simulink model "RoboSoccerSim"  (R2022b)
settings: Solver=ode4  StartTime=0.0  StopTime=inf  FixedStep=0.01  RelTol=1e-3
libraries: dspindex x20
(part 2 of 2)

== stateflow chart RoboSoccerSim/Robot Team Clients 2 (Away)/Subsystem/Away Player Strategy 3 ==
  state InitialState
    en,du:
    if gameSituation.kickConfirmation == true
    robotCommand.kick = false;
    end
    id = 3; % Team1(Home) Robot 1
    shootDistThres = 2500;
    kickableAreaRadius = 20;
    homeGoalPose = [5000, 0];
    awayGoalPose = [-5000, 0];
    homeAttackPositions = [[-2500, 0, 180]; [-1500, 2000, 180]; [-1500, -2000, 180]; [2000, 0, 180]];
    homeDefendPositions = [[1000, 0, 180]; [3000, 2000, 180]; [3000, -2000, 180]; [3500, 0, 180]];
  state ROBOT 1 [group]
    (Strategy for robot 1~3)
  state Attack
    en,du:
    %%calculate the distance to the goal
    teamDistToGoal = [0 0 0 0];
    for idx=1:1:4
    teamDistToGoal(idx) = distTo(gameSituation.robotCurrentPose(idx,1:2), awayGoalPose);
    end
    distToGoal1 = distTo(gameSituation.robotCurrentPose(id,1:2), awayGoalPose);
    %calculate the distance to the ball
    teamDistToBall = [0 0 0 0];
    for idx=1:1:4
    teamDistToBall(idx) = distTo(gameSituation.robotCurrentPose(idx,1:2), ...
    gameSituation.ballCurrentPose(1:2));
    end
    distToBall = distTo(gameSituation.robotCurrentPose(id,1:2), ...
    gameSituation.ballCurrentPose(1:2));
  state Defend
    en,du:
    %%calculate the distance to the home goal
    teamDistToOwnGoal = [0 0 0 0];
    for idx=1:1:4
    teamDistToOwnGoal(idx) = distTo(gameSituation.robotCurrentPose(idx,1:2), homeGoalPose);
    end
    distToOwnGoal = distTo(gameSituation.robotCurrentPose(id,1:2), homeGoalPose);
    for idx=1:1:4
    teamDistToBall(idx) = distTo(gameSituation.robotCurrentPose(idx,1:2), ...
    gameSituation.ballCurrentPose(1:2));
    end
    distToBall = distTo(gameSituation.robotCurrentPose(id,1:2), ...
    gameSituation.ballCurrentPose(1:2));
  state Position
    en,du:
    playerAttackPosition = homeAttackPositions(id, :);
    kickPower = 1;
    kickState = false;
    desiredPosition = playerAttackPosition;
    isdone = true;
  state Shoot
    en,du:
    angleBallGoal = atan2d(awayGoalPose(2) - gameSituation.ballCurrentPose(2), ...
    awayGoalPose(1) - gameSituation.ballCurrentPose(1));
    kickPower = 100;
    kickState = true;
    kickDirection = angleBallGoal;
    xPosition= gameSituation.ballCurrentPose(1) + cosd(180 - angleBallGoal) * kickableAreaRadius;
    yPosition = gameSituation.ballCurrentPose(2) + sind(180 - angleBallGoal) * kickableAreaRadius;
    desiredPosition = [xPosition, yPosition, kickDirection];
    isdone = true;
  state Pass
    en,du:
    [minval,minidx] = min(teamDistToGoal)
    angleBallPlayer = atan2d(gameSituation.robotCurrentPose(minidx, 2) - gameSituation.ballCurrentPose(2), ...
    gameSituation.robotCurrentPose(minidx, 1) - gameSituation.ballCurrentPose(1));
    kickPower = 66;
    kickState = true;
    kickDirection = angleBallPlayer;
    xPosition= gameSituation.ballCurrentPose(1) + cosd(180 - angleBallGoal) * kickableAreaRadius;
    yPosition = gameSituation.ballCurrentPose(2) + sind(180 - angleBallGoal) * kickableAreaRadius;
    desiredPosition = [xPosition, yPosition, kickDirection];
    isdone = true;
  state Dribble
    en,du:
    angleBallGoal = atan2d(awayGoalPose(2) - gameSituation.ballCurrentPose(2), ...
    awayGoalPose(1) - gameSituation.ballCurrentPose(1));
    kickPower = 10;
    %%should be designed as the kickPower = kickPowerCofficent * 100
    %%kickPowerCofficieant should also be calculated by distance
    kickState = true;
    kickDirection = angleBallGoal;
    xPosition= gameSituation.ballCurrentPose(1) + cosd(180 - angleBallGoal) * kickableAreaRadius;
    yPosition = gameSituation.ballCurrentPose(2) + sind(180 - angleBallGoal) * kickableAreaRadius;
    desiredPosition = [xPosition, yPosition, kickDirection];
    isdone = true;
  state Intercept
    en,du:
    angleBallGoal = atan2d(awayGoalPose(2) - gameSituation.ballCurrentPose(2), ...
    awayGoalPose(1) - gameSituation.ballCurrentPose(1));
    kickPower = 50;
    kickState = true;
    kickDirection = angleBallGoal;
    xPosition= gameSituation.ballCurrentPose(1) + cosd(180 - angleBallGoal) * kickableAreaRadius;
    yPosition = gameSituation.ballCurrentPose(2) + sind(180 - angleBallGoal) * kickableAreaRadius;
    desiredPosition = [xPosition, yPosition, kickDirection];
    isdone = true;
  state Formation
    en,du:
    playerDefendPosition = homeDefendPositions(id, :);
    kickPower = 1;
    kickState = false;
    desiredPosition = playerDefendPosition;
    isdone = true;
  state Kick
    state MoveTo1
      en,du:
      isdone = false;
      robotCommand.robotDestinationPose = desiredPosition;
      distToBall = distTo(gameSituation.robotCurrentPose(id,1:2), ...
      gameSituation.ballCurrentPose(1:2));
    state KickTo
      en,du:
      robotCommand.kick = kickState;
      robotCommand.kickProperty = kickPower;
      isdone = true;
    MoveTo1 -> KickTo [order 1] : [distToBall <= kickableAreaRadius+5]
  MoveTo1 -> InitialState [order 2] : [after(2,sec)]
  KickTo -> InitialState : [after(5,sec)]
  (default) -> InitialState
  InitialState -> Attack [order 2] : [gameSituation.ballLastCommandBy(1) == 2]
  InitialState -> Defend [order 1] : [gameSituation.ballLastCommandBy(1) == 1]
  Attack -> Position [order 1] : [distToBall ~= min(teamDistToBall)]
  Defend -> Intercept [order 1] : [distToBall ~= max(teamDistToBall)]
  Defend -> Formation [order 2] : [distToBall == max(teamDistToBall)]
  Attack -> Pass [order 3] : [distToGoal1 ~= min(teamDistToGoal)&& distToBall == min(teamDistToBall)]
  Attack -> Dribble [order 4] : [distToBall == min(teamDistToBall) && distToGoal1 == min(teamDistToGoal) && distToGoal1 > shootDistThres]
  Attack -> Shoot [order 2] : [distToBall == min(teamDistToBall) && distToGoal1 == min(teamDistToGoal) && distToGoal1 < shootDistThres]
  Intercept -> MoveTo1 : [isdone]
  Formation -> MoveTo1 : [isdone]
  Pass -> MoveTo1 : [isdone]
  Dribble -> MoveTo1 : [isdone]
  Shoot -> MoveTo1 : [isdone]
  Position -> MoveTo1 : [isdone]
  data: robotPosition function_input; goalPosition function_input; dist function_output; awayGoalPose local =[0 0]; homeGoalPose local =[0 0]; id local =1; idx local; angleBallGoal local =0; desiredPosition local =[0 0 0]; distToOwnGoal local =0; kickDirection local =0; kickPower local =0; kickState local =false; minidx local; playerDefendPosition local =[0 0 0]; teamDistToGoal local =[0 0 0 0]; teamDistToOwnGoal local =[0 0 0 0]; minval local; isdone local boolean =false; playerAttackPosition local =[0 0 0]; shootDistThres local =0; gameSituation input Bus: gameSituation; kickableAreaRadius local =0; distToGoal1 local =0; angleBallPlayer local =0; robotCommand output Bus: robotCommand; distToBall local =0; teamDistToBall local =[0 0 0 0]; homeAttackPositions local =[0 0 0;0 0 0;0 0 0;0 0 0]; homeDefendPositions local =[0 0 0;0 0 0;0 0 0;0 0 0]; xPosition local; yPosition local
  function dist = distTo(robotPosition,goalPosition):
    | function dist = distTo(robotPosition,goalPosition)
    |     dist = norm(robotPosition - goalPosition);
    | end

== stateflow chart RoboSoccerSim/Robot Team Clients 1 (Home)/Subsystem/Home Player Strategy 1 ==
  state InitialState
    en,du:
    if gameSituation.kickConfirmation == true
    robotCommand.kick = false;
    end
    id = 1; % Team1(Home) Robot 1
    shootDistThres = 2500;
    kickableAreaRadius = 20;
    homeGoalPose = [-5000, 0];
    awayGoalPose = [5000, 0];
    homeAttackPositions = [[2500, 0, 0]; [1500, 2000, 0]; [1500, -2000, 0]; [-2000, 0, 0]];
    homeDefendPositions = [[-1000, 0, 0]; [-3000, 2000, 0]; [-3000, -2000, 0]; [-3500, 0, 0]];
  state ROBOT 1 [group]
    (Strategy for robot 1~3)
  state Attack
    en,du:
    %%calculate the distance to the goal
    teamDistToGoal = [0 0 0 0];
    for idx=1:1:4
    teamDistToGoal(idx) = distTo(gameSituation.robotCurrentPose(idx,1:2), awayGoalPose);
    end
    distToGoal1 = distTo(gameSituation.robotCurrentPose(id,1:2), awayGoalPose);
    %calculate the distance to the ball
    teamDistToBall = [0 0 0 0];
    for idx=1:1:4
    teamDistToBall(idx) = distTo(gameSituation.robotCurrentPose(idx,1:2), ...
    gameSituation.ballCurrentPose(1:2));
    end
    distToBall = distTo(gameSituation.robotCurrentPose(id,1:2), ...
    gameSituation.ballCurrentPose(1:2));
  state Defend
    en,du:
    %%calculate the distance to the home goal
    teamDistToOwnGoal = [0 0 0 0];
    for idx=1:1:4
    teamDistToOwnGoal(idx) = distTo(gameSituation.robotCurrentPose(idx,1:2), homeGoalPose);
    end
    distToOwnGoal = distTo(gameSituation.robotCurrentPose(id,1:2), homeGoalPose);
    for idx=1:1:4
    teamDistToBall(idx) = distTo(gameSituation.robotCurrentPose(idx,1:2), ...
    gameSituation.ballCurrentPose(1:2));
    end
    distToBall = distTo(gameSituation.robotCurrentPose(id,1:2), ...
    gameSituation.ballCurrentPose(1:2));
  state Position
    en,du:
    playerAttackPosition = homeAttackPositions(id, :);
    kickPower = 1;
    kickState = false;
    desiredPosition = playerAttackPosition;
    isdone = true;
  state Shoot
    en,du:
    angleBallGoal = atan2d(awayGoalPose(2) - gameSituation.ballCurrentPose(2), ...
    awayGoalPose(1) - gameSituation.ballCurrentPose(1));
    kickPower = 100;
    kickState = true;
    kickDirection = angleBallGoal;
    xPosition= gameSituation.ballCurrentPose(1) + cosd(180 - angleBallGoal) * kickableAreaRadius;
    yPosition = gameSituation.ballCurrentPose(2) + sind(180 - angleBallGoal) * kickableAreaRadius;
    desiredPosition = [xPosition, yPosition, kickDirection];
    isdone = true;
  state Pass
    en,du:
    [minval,minidx] = min(teamDistToGoal)
    angleBallPlayer = atan2d(gameSituation.robotCurrentPose(minidx, 2) - gameSituation.ballCurrentPose(2), ...
    gameSituation.robotCurrentPose(minidx, 1) - gameSituation.ballCurrentPose(1));
    kickPower = 66;
    kickState = true;
    kickDirection = angleBallPlayer;
    xPosition= gameSituation.ballCurrentPose(1) + cosd(180 - angleBallGoal) * kickableAreaRadius;
    yPosition = gameSituation.ballCurrentPose(2) + sind(180 - angleBallGoal) * kickableAreaRadius;
    desiredPosition = [xPosition, yPosition, kickDirection];
    isdone = true;
  state Dribble
    en,du:
    angleBallGoal = atan2d(awayGoalPose(2) - gameSituation.ballCurrentPose(2), ...
    awayGoalPose(1) - gameSituation.ballCurrentPose(1));
    kickPower = 20;
    %%should be designed as the kickPower = kickPowerCofficent * 100
    %%kickPowerCofficieant should also be calculated by distance
    kickState = true;
    kickDirection = angleBallGoal;
    xPosition= gameSituation.ballCurrentPose(1) + cosd(180 - angleBallGoal) * kickableAreaRadius;
    yPosition = gameSituation.ballCurrentPose(2) + sind(180 - angleBallGoal) * kickableAreaRadius;
    desiredPosition = [xPosition, yPosition, kickDirection];
    isdone = true;
  state Intercept
    en,du:
    angleBallGoal = atan2d(awayGoalPose(2) - gameSituation.ballCurrentPose(2), ...
    awayGoalPose(1) - gameSituation.ballCurrentPose(1));
    kickPower = 50;
    kickState = true;
    kickDirection = angleBallGoal;
    xPosition= gameSituation.ballCurrentPose(1) + cosd(180 - angleBallGoal) * kickableAreaRadius;
    yPosition = gameSituation.ballCurrentPose(2) + sind(180 - angleBallGoal) * kickableAreaRadius;
    desiredPosition = [xPosition, yPosition, kickDirection];
    isdone = true;
  state Formation
    en,du:
    playerDefendPosition = homeDefendPositions(id, :);
    kickPower = 1;
    kickState = false;
    desiredPosition = playerDefendPosition;
    isdone = true;
  state Kick
    state MoveTo1
      en,du:
      isdone = false;
      robotCommand.robotDestinationPose = desiredPosition;
      distToBall = distTo(gameSituation.robotCurrentPose(id,1:2), ...
      gameSituation.ballCurrentPose(1:2));
    state KickTo
      en,du:
      robotCommand.kick = kickState;
      robotCommand.kickProperty = kickPower;
      isdone = true;
    MoveTo1 -> KickTo [order 1] : [distToBall <= kickableAreaRadius+5]
  MoveTo1 -> InitialState [order 2] : [after(2,sec)]
  KickTo -> InitialState : [after(5,sec)]
  (default) -> InitialState
  InitialState -> Attack [order 2] : [gameSituation.ballLastCommandBy(1) == 1]
  InitialState -> Defend [order 1] : [gameSituation.ballLastCommandBy(1) == 2]
  Attack -> Position [order 1] : [distToBall ~= min(teamDistToBall)]
  Defend -> Intercept [order 1] : [distToBall ~= max(teamDistToBall)]
  Defend -> Formation [order 2] : [distToBall == max(teamDistToBall)]
  Attack -> Pass [order 3] : [distToGoal1 ~= min(teamDistToGoal)&& distToBall == min(teamDistToBall)]
  Attack -> Dribble [order 4] : [distToBall == min(teamDistToBall) && distToGoal1 == min(teamDistToGoal) && distToGoal1 > shootDistThres]
  Attack -> Shoot [order 2] : [distToBall == min(teamDistToBall) && distToGoal1 == min(teamDistToGoal) && distToGoal1 < shootDistThres]
  Intercept -> MoveTo1 : [isdone]
  Formation -> MoveTo1 : [isdone]
  Pass -> MoveTo1 : [isdone]
  Dribble -> MoveTo1 : [isdone]
  Shoot -> MoveTo1 : [isdone]
  Position -> MoveTo1 : [isdone]
  data: robotPosition function_input; goalPosition function_input; dist function_output; awayGoalPose local =[0 0]; homeGoalPose local =[0 0]; id local =1; idx local; angleBallGoal local =0; desiredPosition local =[0 0 0]; distToOwnGoal local =0; kickDirection local =0; kickPower local =0; kickState local =false; minidx local; playerDefendPosition local =[0 0 0]; teamDistToGoal local =[0 0 0 0]; teamDistToOwnGoal local =[0 0 0 0]; minval local; isdone local boolean =false; playerAttackPosition local =[0 0 0]; shootDistThres local =0; gameSituation input Bus: gameSituation; kickableAreaRadius local =0; distToGoal1 local =0; angleBallPlayer local =0; robotCommand output Bus: robotCommand; distToBall local =0; teamDistToBall local =[0 0 0 0]; homeAttackPositions local =[0 0 0;0 0 0;0 0 0;0 0 0]; homeDefendPositions local =[0 0 0;0 0 0;0 0 0;0 0 0]; xPosition local; yPosition local
  function dist = distTo(robotPosition,goalPosition):
    | function dist = distTo(robotPosition,goalPosition)
    |     dist = norm(robotPosition - goalPosition);
    | end

== stateflow chart RoboSoccerSim/Robot Team Clients 1 (Home)/Subsystem/Home Player Strategy 2 ==
  state InitialState
    en,du:
    if gameSituation.kickConfirmation == true
    robotCommand.kick = false;
    end
    id = 2; % Team1(Home) Robot 1
    shootDistThres = 2500;
    kickableAreaRadius = 20;
    homeGoalPose = [-5000, 0];
    awayGoalPose = [5000, 0];
    homeAttackPositions = [[2500, 0, 0]; [1500, 2000, 0]; [1500, -2000, 0]; [-2000, 0, 0]];
    homeDefendPositions = [[-1000, 0, 0]; [-3000, 2000, 0]; [-3000, -2000, 0]; [-3500, 0, 0]];
  state ROBOT 1 [group]
    (Strategy for robot 1~3)
  state Attack
    en,du:
    %%calculate the distance to the goal
    teamDistToGoal = [0 0 0 0];
    for idx=1:1:4
    teamDistToGoal(idx) = distTo(gameSituation.robotCurrentPose(idx,1:2), awayGoalPose);
    end
    distToGoal1 = distTo(gameSituation.robotCurrentPose(id,1:2), awayGoalPose);
    %calculate the distance to the ball
    teamDistToBall = [0 0 0 0];
    for idx=1:1:4
    teamDistToBall(idx) = distTo(gameSituation.robotCurrentPose(idx,1:2), ...
    gameSituation.ballCurrentPose(1:2));
    end
    distToBall = distTo(gameSituation.robotCurrentPose(id,1:2), ...
    gameSituation.ballCurrentPose(1:2));
  state Defend
    en,du:
    %%calculate the distance to the home goal
    teamDistToOwnGoal = [0 0 0 0];
    for idx=1:1:4
    teamDistToOwnGoal(idx) = distTo(gameSituation.robotCurrentPose(idx,1:2), homeGoalPose);
    end
    distToOwnGoal = distTo(gameSituation.robotCurrentPose(id,1:2), homeGoalPose);
    for idx=1:1:4
    teamDistToBall(idx) = distTo(gameSituation.robotCurrentPose(idx,1:2), ...
    gameSituation.ballCurrentPose(1:2));
    end
    distToBall = distTo(gameSituation.robotCurrentPose(id,1:2), ...
    gameSituation.ballCurrentPose(1:2));
  state Position
    en,du:
    playerAttackPosition = homeAttackPositions(id, :);
    kickPower = 1;
    kickState = false;
    desiredPosition = playerAttackPosition;
    isdone = true;
  state Shoot
    en,du:
    angleBallGoal = atan2d(awayGoalPose(2) - gameSituation.ballCurrentPose(2), ...
    awayGoalPose(1) - gameSituation.ballCurrentPose(1));
    kickPower = 100;
    kickState = true;
    kickDirection = angleBallGoal;
    xPosition= gameSituation.ballCurrentPose(1) + cosd(180 - angleBallGoal) * kickableAreaRadius;
    yPosition = gameSituation.ballCurrentPose(2) + sind(180 - angleBallGoal) * kickableAreaRadius;
    desiredPosition = [xPosition, yPosition, kickDirection];
    isdone = true;
  state Pass
    en,du:
    [minval,minidx] = min(teamDistToGoal)
    angleBallPlayer = atan2d(gameSituation.robotCurrentPose(minidx, 2) - gameSituation.ballCurrentPose(2), ...
    gameSituation.robotCurrentPose(minidx, 1) - gameSituation.ballCurrentPose(1));
    kickPower = 66;
    kickState = true;
    kickDirection = angleBallPlayer;
    xPosition= gameSituation.ballCurrentPose(1) + cosd(180 - angleBallGoal) * kickableAreaRadius;
    yPosition = gameSituation.ballCurrentPose(2) + sind(180 - angleBallGoal) * kickableAreaRadius;
    desiredPosition = [xPosition, yPosition, kickDirection];
    isdone = true;
  state Dribble
    en,du:
    angleBallGoal = atan2d(awayGoalPose(2) - gameSituation.ballCurrentPose(2), ...
    awayGoalPose(1) - gameSituation.ballCurrentPose(1));
    kickPower = 20;
    %%should be designed as the kickPower = kickPowerCofficent * 100
    %%kickPowerCofficieant should also be calculated by distance
    kickState = true;
    kickDirection = angleBallGoal;
    xPosition= gameSituation.ballCurrentPose(1) + cosd(180 - angleBallGoal) * kickableAreaRadius;
    yPosition = gameSituation.ballCurrentPose(2) + sind(180 - angleBallGoal) * kickableAreaRadius;
    desiredPosition = [xPosition, yPosition, kickDirection];
    isdone = true;
  state Intercept
    en,du:
    angleBallGoal = atan2d(awayGoalPose(2) - gameSituation.ballCurrentPose(2), ...
    awayGoalPose(1) - gameSituation.ballCurrentPose(1));
    kickPower = 50;
    kickState = true;
    kickDirection = angleBallGoal;
    xPosition= gameSituation.ballCurrentPose(1) + cosd(180 - angleBallGoal) * kickableAreaRadius;
    yPosition = gameSituation.ballCurrentPose(2) + sind(180 - angleBallGoal) * kickableAreaRadius;
    desiredPosition = [xPosition, yPosition, kickDirection];
    isdone = true;
  state Formation
    en,du:
    playerDefendPosition = homeDefendPositions(id, :);
    kickPower = 1;
    kickState = false;
    desiredPosition = playerDefendPosition;
    isdone = true;
  state Kick
    state MoveTo1
      en,du:
      isdone = false;
      robotCommand.robotDestinationPose = desiredPosition;
      distToBall = distTo(gameSituation.robotCurrentPose(id,1:2), ...
      gameSituation.ballCurrentPose(1:2));
    state KickTo
      en,du:
      robotCommand.kick = kickState;
      robotCommand.kickProperty = kickPower;
      isdone = true;
    MoveTo1 -> KickTo [order 1] : [distToBall <= kickableAreaRadius+5]
  MoveTo1 -> InitialState [order 2] : [after(2,sec)]
  KickTo -> InitialState : [after(5,sec)]
  (default) -> InitialState
  InitialState -> Attack [order 2] : [gameSituation.ballLastCommandBy(1) == 1]
  InitialState -> Defend [order 1] : [gameSituation.ballLastCommandBy(1) == 2]
  Attack -> Position [order 1] : [distToBall ~= min(teamDistToBall)]
  Defend -> Intercept [order 1] : [distToBall ~= max(teamDistToBall)]
  Defend -> Formation [order 2] : [distToBall == max(teamDistToBall)]
  Attack -> Pass [order 3] : [distToGoal1 ~= min(teamDistToGoal)&& distToBall == min(teamDistToBall)]
  Attack -> Dribble [order 4] : [distToBall == min(teamDistToBall) && distToGoal1 == min(teamDistToGoal) && distToGoal1 > shootDistThres]
  Attack -> Shoot [order 2] : [distToBall == min(teamDistToBall) && distToGoal1 == min(teamDistToGoal) && distToGoal1 < shootDistThres]
  Intercept -> MoveTo1 : [isdone]
  Formation -> MoveTo1 : [isdone]
  Pass -> MoveTo1 : [isdone]
  Dribble -> MoveTo1 : [isdone]
  Shoot -> MoveTo1 : [isdone]
  Position -> MoveTo1 : [isdone]
  data: robotPosition function_input; goalPosition function_input; dist function_output; awayGoalPose local =[0 0]; homeGoalPose local =[0 0]; id local =1; idx local; angleBallGoal local =0; desiredPosition local =[0 0 0]; distToOwnGoal local =0; kickDirection local =0; kickPower local =0; kickState local =false; minidx local; playerDefendPosition local =[0 0 0]; teamDistToGoal local =[0 0 0 0]; teamDistToOwnGoal local =[0 0 0 0]; minval local; isdone local boolean =false; playerAttackPosition local =[0 0 0]; shootDistThres local =0; gameSituation input Bus: gameSituation; kickableAreaRadius local =0; distToGoal1 local =0; angleBallPlayer local =0; robotCommand output Bus: robotCommand; distToBall local =0; teamDistToBall local =[0 0 0 0]; homeAttackPositions local =[0 0 0;0 0 0;0 0 0;0 0 0]; homeDefendPositions local =[0 0 0;0 0 0;0 0 0;0 0 0]; xPosition local; yPosition local
  function dist = distTo(robotPosition,goalPosition):
    | function dist = distTo(robotPosition,goalPosition)
    |     dist = norm(robotPosition - goalPosition);
    | end

== stateflow chart RoboSoccerSim/Robot Team Clients 1 (Home)/Subsystem/Home Player Strategy 3 ==
  state InitialState
    en,du:
    if gameSituation.kickConfirmation == true
    robotCommand.kick = false;
    end
    id = 3; % Team1(Home) Robot 1
    shootDistThres = 2500;
    kickableAreaRadius = 20;
    homeGoalPose = [-5000, 0];
    awayGoalPose = [5000, 0];
    homeAttackPositions = [[2500, 0, 0]; [1500, 2000, 0]; [1500, -2000, 0]; [-2000, 0, 0]];
    homeDefendPositions = [[-1000, 0, 0]; [-3000, 2000, 0]; [-3000, -2000, 0]; [-3500, 0, 0]];
  state ROBOT 1 [group]
    (Strategy for robot 1~3)
  state Attack
    en,du:
    %%calculate the distance to the goal
    teamDistToGoal = [0 0 0 0];
    for idx=1:1:4
    teamDistToGoal(idx) = distTo(gameSituation.robotCurrentPose(idx,1:2), awayGoalPose);
    end
    distToGoal1 = distTo(gameSituation.robotCurrentPose(id,1:2), awayGoalPose);
    %calculate the distance to the ball
    teamDistToBall = [0 0 0 0];
    for idx=1:1:4
    teamDistToBall(idx) = distTo(gameSituation.robotCurrentPose(idx,1:2), ...
    gameSituation.ballCurrentPose(1:2));
    end
    distToBall = distTo(gameSituation.robotCurrentPose(id,1:2), ...
    gameSituation.ballCurrentPose(1:2));
  state Defend
    en,du:
    %%calculate the distance to the home goal
    teamDistToOwnGoal = [0 0 0 0];
    for idx=1:1:4
    teamDistToOwnGoal(idx) = distTo(gameSituation.robotCurrentPose(idx,1:2), homeGoalPose);
    end
    distToOwnGoal = distTo(gameSituation.robotCurrentPose(id,1:2), homeGoalPose);
    for idx=1:1:4
    teamDistToBall(idx) = distTo(gameSituation.robotCurrentPose(idx,1:2), ...
    gameSituation.ballCurrentPose(1:2));
    end
    distToBall = distTo(gameSituation.robotCurrentPose(id,1:2), ...
    gameSituation.ballCurrentPose(1:2));
  state Position
    en,du:
    playerAttackPosition = homeAttackPositions(id, :);
    kickPower = 1;
    kickState = false;
    desiredPosition = playerAttackPosition;
    isdone = true;
  state Shoot
    en,du:
    angleBallGoal = atan2d(awayGoalPose(2) - gameSituation.ballCurrentPose(2), ...
    awayGoalPose(1) - gameSituation.ballCurrentPose(1));
    kickPower = 100;
    kickState = true;
    kickDirection = angleBallGoal;
    xPosition= gameSituation.ballCurrentPose(1) + cosd(180 - angleBallGoal) * kickableAreaRadius;
    yPosition = gameSituation.ballCurrentPose(2) + sind(180 - angleBallGoal) * kickableAreaRadius;
    desiredPosition = [xPosition, yPosition, kickDirection];
    isdone = true;
  state Pass
    en,du:
    [minval,minidx] = min(teamDistToGoal)
    angleBallPlayer = atan2d(gameSituation.robotCurrentPose(minidx, 2) - gameSituation.ballCurrentPose(2), ...
    gameSituation.robotCurrentPose(minidx, 1) - gameSituation.ballCurrentPose(1));
    kickPower = 66;
    kickState = true;
    kickDirection = angleBallPlayer;
    xPosition= gameSituation.ballCurrentPose(1) + cosd(180 - angleBallGoal) * kickableAreaRadius;
    yPosition = gameSituation.ballCurrentPose(2) + sind(180 - angleBallGoal) * kickableAreaRadius;
    desiredPosition = [xPosition, yPosition, kickDirection];
    isdone = true;
  state Dribble
    en,du:
    angleBallGoal = atan2d(awayGoalPose(2) - gameSituation.ballCurrentPose(2), ...
    awayGoalPose(1) - gameSituation.ballCurrentPose(1));
    kickPower = 20;
    %%should be designed as the kickPower = kickPowerCofficent * 100
    %%kickPowerCofficieant should also be calculated by distance
    kickState = true;
    kickDirection = angleBallGoal;
    xPosition= gameSituation.ballCurrentPose(1) + cosd(180 - angleBallGoal) * kickableAreaRadius;
    yPosition = gameSituation.ballCurrentPose(2) + sind(180 - angleBallGoal) * kickableAreaRadius;
    desiredPosition = [xPosition, yPosition, kickDirection];
    isdone = true;
  state Intercept
    en,du:
    angleBallGoal = atan2d(awayGoalPose(2) - gameSituation.ballCurrentPose(2), ...
    awayGoalPose(1) - gameSituation.ballCurrentPose(1));
    kickPower = 50;
    kickState = true;
    kickDirection = angleBallGoal;
    xPosition= gameSituation.ballCurrentPose(1) + cosd(180 - angleBallGoal) * kickableAreaRadius;
    yPosition = gameSituation.ballCurrentPose(2) + sind(180 - angleBallGoal) * kickableAreaRadius;
    desiredPosition = [xPosition, yPosition, kickDirection];
    isdone = true;
  state Formation
    en,du:
    playerDefendPosition = homeDefendPositions(id, :);
    kickPower = 1;
    kickState = false;
    desiredPosition = playerDefendPosition;
    isdone = true;
  state Kick
    state MoveTo1
      en,du:
      isdone = false;
      robotCommand.robotDestinationPose = desiredPosition;
      distToBall = distTo(gameSituation.robotCurrentPose(id,1:2), ...
      gameSituation.ballCurrentPose(1:2));
    state KickTo
      en,du:
      robotCommand.kick = kickState;
      robotCommand.kickProperty = kickPower;
      isdone = true;
    MoveTo1 -> KickTo [order 1] : [distToBall <= kickableAreaRadius+5]
  MoveTo1 -> InitialState [order 2] : [after(2,sec)]
  KickTo -> InitialState : [after(5,sec)]
  (default) -> InitialState
  InitialState -> Attack [order 2] : [gameSituation.ballLastCommandBy(1) == 1]
  InitialState -> Defend [order 1] : [gameSituation.ballLastCommandBy(1) == 2]
  Attack -> Position [order 1] : [distToBall ~= min(teamDistToBall)]
  Defend -> Intercept [order 1] : [distToBall ~= max(teamDistToBall)]
  Defend -> Formation [order 2] : [distToBall == max(teamDistToBall)]
  Attack -> Pass [order 3] : [distToGoal1 ~= min(teamDistToGoal)&& distToBall == min(teamDistToBall)]
  Attack -> Dribble [order 4] : [distToBall == min(teamDistToBall) && distToGoal1 == min(teamDistToGoal) && distToGoal1 > shootDistThres]
  Attack -> Shoot [order 2] : [distToBall == min(teamDistToBall) && distToGoal1 == min(teamDistToGoal) && distToGoal1 < shootDistThres]
  Intercept -> MoveTo1 : [isdone]
  Formation -> MoveTo1 : [isdone]
  Pass -> MoveTo1 : [isdone]
  Dribble -> MoveTo1 : [isdone]
  Shoot -> MoveTo1 : [isdone]
  Position -> MoveTo1 : [isdone]
  data: robotPosition function_input; goalPosition function_input; dist function_output; awayGoalPose local =[0 0]; homeGoalPose local =[0 0]; id local =1; idx local; angleBallGoal local =0; desiredPosition local =[0 0 0]; distToOwnGoal local =0; kickDirection local =0; kickPower local =0; kickState local =false; minidx local; playerDefendPosition local =[0 0 0]; teamDistToGoal local =[0 0 0 0]; teamDistToOwnGoal local =[0 0 0 0]; minval local; isdone local boolean =false; playerAttackPosition local =[0 0 0]; shootDistThres local =0; gameSituation input Bus: gameSituation; kickableAreaRadius local =0; distToGoal1 local =0; angleBallPlayer local =0; robotCommand output Bus: robotCommand; distToBall local =0; teamDistToBall local =[0 0 0 0]; homeAttackPositions local =[0 0 0;0 0 0;0 0 0;0 0 0]; homeDefendPositions local =[0 0 0;0 0 0;0 0 0;0 0 0]; xPosition local; yPosition local
  function dist = distTo(robotPosition,goalPosition):
    | function dist = distTo(robotPosition,goalPosition)
    |     dist = norm(robotPosition - goalPosition);
    | end

== stateflow chart RoboSoccerSim/Robot Team Clients 1 (Home)/Subsystem/Home Player Strategy 4 ==
  state InitialState
    en,du:
    if gameSituation.kickConfirmation == true
    robotCommand.kick = false;
    end
    id = 4; % Team1(Home) Robot 1
    shootDistThres = 2500;
    kickableAreaRadius = 100;
    homeGoalPose = [-5000, 0];
    awayGoalPose = [5000, 0];
    homeAttackPositions = [[2500, 0, 0]; [1500, 2000, 0]; [1500, -2000, 0]; [-2000, 0, 0]];
    homeDefendPositions = [[-1000, 0, 0]; [-3000, 2000, 0]; [-3000, -2000, 0]; [-3500, 0, 0]];
  state ROBOT 1 [group]
    (Strategy for robot 1~3)
  state Attack
    en,du:
    %%calculate the distance to the goal
    teamDistToGoal = [0 0 0 0];
    for idx=1:1:4
    teamDistToGoal(idx) = distTo(gameSituation.robotCurrentPose(idx,1:2), awayGoalPose);
    end
    distToGoal1 = distTo(gameSituation.robotCurrentPose(id,1:2), awayGoalPose);
    %calculate the distance to the ball
    teamDistToBall = [0 0 0 0];
    for idx=1:1:4
    teamDistToBall(idx) = distTo(gameSituation.robotCurrentPose(idx,1:2), ...
    gameSituation.ballCurrentPose(1:2));
    end
    distToBall = distTo(gameSituation.robotCurrentPose(id,1:2), ...
    gameSituation.ballCurrentPose(1:2));
  state Defend
    en,du:
    %%calculate the distance to the home goal
    teamDistToOwnGoal = [0 0 0 0];
    for idx=1:1:4
    teamDistToOwnGoal(idx) = distTo(gameSituation.robotCurrentPose(idx,1:2), homeGoalPose);
    end
    distToOwnGoal = distTo(gameSituation.robotCurrentPose(id,1:2), homeGoalPose);
    for idx=1:1:4
    teamDistToBall(idx) = distTo(gameSituation.robotCurrentPose(idx,1:2), ...
    gameSituation.ballCurrentPose(1:2));
    end
    distToBall = distTo(gameSituation.robotCurrentPose(id,1:2), ...
    gameSituation.ballCurrentPose(1:2));
  state Position
    en,du:
    playerAttackPosition = homeAttackPositions(id, :);
    kickPower = 1;
    kickState = false;
    desiredPosition = playerAttackPosition;
    isdone = true;
  state Shoot
    en,du:
    angleBallGoal = atan2d(awayGoalPose(2) - gameSituation.ballCurrentPose(2), ...
    awayGoalPose(1) - gameSituation.ballCurrentPose(1));
    kickPower = 100;
    kickState = true;
    kickDirection = angleBallGoal;
    xPosition= gameSituation.ballCurrentPose(1) + cosd(180 - angleBallGoal) * kickableAreaRadius;
    yPosition = gameSituation.ballCurrentPose(2) + sind(180 - angleBallGoal) * kickableAreaRadius;
    desiredPosition = [xPosition, yPosition, kickDirection];
    isdone = true;
  state Pass
    en,du:
    [minval,minidx] = min(teamDistToGoal)
    angleBallPlayer = atan2d(gameSituation.robotCurrentPose(minidx, 2) - gameSituation.ballCurrentPose(2), ...
    gameSituation.robotCurrentPose(minidx, 1) - gameSituation.ballCurrentPose(1));
    kickPower = 66;
    kickState = true;
    kickDirection = angleBallPlayer;
    xPosition= gameSituation.ballCurrentPose(1) + cosd(180 - angleBallGoal) * kickableAreaRadius;
    yPosition = gameSituation.ballCurrentPose(2) + sind(180 - angleBallGoal) * kickableAreaRadius;
    desiredPosition = [xPosition, yPosition, kickDirection];
    isdone = true;
  state Dribble
    en,du:
    angleBallGoal = atan2d(awayGoalPose(2) - gameSituation.ballCurrentPose(2), ...
    awayGoalPose(1) - gameSituation.ballCurrentPose(1));
    kickPower = 20;
    %%should be designed as the kickPower = kickPowerCofficent * 100
    %%kickPowerCofficieant should also be calculated by distance
    kickState = true;
    kickDirection = angleBallGoal;
    xPosition= gameSituation.ballCurrentPose(1) + cosd(180 - angleBallGoal) * kickableAreaRadius;
    yPosition = gameSituation.ballCurrentPose(2) + sind(180 - angleBallGoal) * kickableAreaRadius;
    desiredPosition = [xPosition, yPosition, kickDirection];
    isdone = true;
  state Intercept
    en,du:
    angleBallGoal = atan2d(awayGoalPose(2) - gameSituation.ballCurrentPose(2), ...
    awayGoalPose(1) - gameSituation.ballCurrentPose(1));
    kickPower = 50;
    kickState = true;
    kickDirection = angleBallGoal;
    xPosition= gameSituation.ballCurrentPose(1) + cosd(180 - angleBallGoal) * kickableAreaRadius;
    yPosition = gameSituation.ballCurrentPose(2) + sind(180 - angleBallGoal) * kickableAreaRadius;
    desiredPosition = [xPosition, yPosition, kickDirection];
    isdone = true;
  state Formation
    en,du:
    playerDefendPosition = homeDefendPositions(id, :);
    kickPower = 1;
    kickState = false;
    desiredPosition = playerDefendPosition;
    isdone = true;
  state Kick
    state MoveTo1
      en,du:
      isdone = false;
      robotCommand.robotDestinationPose = desiredPosition;
      distToBall = distTo(gameSituation.robotCurrentPose(id,1:2), ...
      gameSituation.ballCurrentPose(1:2));
    state KickTo
      en,du:
      robotCommand.kick = kickState;
      robotCommand.kickProperty = kickPower;
      isdone = true;
    MoveTo1 -> KickTo [order 1] : [distToBall <= kickableAreaRadius+5]
  MoveTo1 -> InitialState [order 2] : [after(2,sec)]
  KickTo -> InitialState : [after(5,sec)]
  (default) -> InitialState
  InitialState -> Attack [order 2] : [gameSituation.ballLastCommandBy(1) == 1]
  InitialState -> Defend [order 1] : [gameSituation.ballLastCommandBy(1) == 2]
  Attack -> Position [order 1] : [distToBall ~= min(teamDistToBall)]
  Defend -> Intercept [order 1] : [distToBall ~= max(teamDistToBall)]
  Defend -> Formation [order 2] : [distToBall == max(teamDistToBall)]
  Attack -> Pass [order 3] : [distToGoal1 ~= min(teamDistToGoal)&& distToBall == min(teamDistToBall)]
  Attack -> Dribble [order 4] : [distToBall == min(teamDistToBall) && distToGoal1 == min(teamDistToGoal) && distToGoal1 > shootDistThres]
  Attack -> Shoot [order 2] : [distToBall == min(teamDistToBall) && distToGoal1 == min(teamDistToGoal) && distToGoal1 < shootDistThres]
  Intercept -> MoveTo1 : [isdone]
  Formation -> MoveTo1 : [isdone]
  Pass -> MoveTo1 : [isdone]
  Dribble -> MoveTo1 : [isdone]
  Shoot -> MoveTo1 : [isdone]
  Position -> MoveTo1 : [isdone]
  data: robotPosition function_input; goalPosition function_input; dist function_output; awayGoalPose local =[0 0]; homeGoalPose local =[0 0]; id local =1; idx local; angleBallGoal local =0; desiredPosition local =[0 0 0]; distToOwnGoal local =0; kickDirection local =0; kickPower local =0; kickState local =false; minidx local; playerDefendPosition local =[0 0 0]; teamDistToGoal local =[0 0 0 0]; teamDistToOwnGoal local =[0 0 0 0]; minval local; isdone local boolean =false; playerAttackPosition local =[0 0 0]; shootDistThres local =0; gameSituation input Bus: gameSituation; kickableAreaRadius local =0; distToGoal1 local =0; angleBallPlayer local =0; robotCommand output Bus: robotCommand; distToBall local =0; teamDistToBall local =[0 0 0 0]; homeAttackPositions local =[0 0 0;0 0 0;0 0 0;0 0 0]; homeDefendPositions local =[0 0 0;0 0 0;0 0 0;0 0 0]; xPosition local; yPosition local
  function dist = distTo(robotPosition,goalPosition):
    | function dist = distTo(robotPosition,goalPosition)
    |     dist = norm(robotPosition - goalPosition);
    | end

== stateflow chart RoboSoccerSim/Robot Team Clients 2 (Away)/Subsystem/Away Player Strategy 4 ==
  state InitialState
    en,du:
    if gameSituation.kickConfirmation == true
    robotCommand.kick = false;
    end
    id = 4; % Team1(Home) Robot 1
    shootDistThres = 2500;
    kickableAreaRadius = 100;
    homeGoalPose = [5000, 0];
    awayGoalPose = [-5000, 0];
    homeAttackPositions = [[-2500, 0, 180]; [-1500, 2000, 180]; [-1500, -2000, 180]; [2000, 0, 180]];
    homeDefendPositions = [[1000, 0, 180]; [3000, 2000, 180]; [3000, -2000, 180]; [3500, 0, 180]];
  state ROBOT 1 [group]
    (Strategy for robot 1~3)
  state Attack
    en,du:
    %%calculate the distance to the goal
    teamDistToGoal = [0 0 0 0];
    for idx=1:1:4
    teamDistToGoal(idx) = distTo(gameSituation.robotCurrentPose(idx,1:2), awayGoalPose);
    end
    distToGoal1 = distTo(gameSituation.robotCurrentPose(id,1:2), awayGoalPose);
    %calculate the distance to the ball
    teamDistToBall = [0 0 0 0];
    for idx=1:1:4
    teamDistToBall(idx) = distTo(gameSituation.robotCurrentPose(idx,1:2), ...
    gameSituation.ballCurrentPose(1:2));
    end
    distToBall = distTo(gameSituation.robotCurrentPose(id,1:2), ...
    gameSituation.ballCurrentPose(1:2));
  state Defend
    en,du:
    %%calculate the distance to the home goal
    teamDistToOwnGoal = [0 0 0 0];
    for idx=1:1:4
    teamDistToOwnGoal(idx) = distTo(gameSituation.robotCurrentPose(idx,1:2), homeGoalPose);
    end
    distToOwnGoal = distTo(gameSituation.robotCurrentPose(id,1:2), homeGoalPose);
    for idx=1:1:4
    teamDistToBall(idx) = distTo(gameSituation.robotCurrentPose(idx,1:2), ...
    gameSituation.ballCurrentPose(1:2));
    end
    distToBall = distTo(gameSituation.robotCurrentPose(id,1:2), ...
    gameSituation.ballCurrentPose(1:2));
  state Position
    en,du:
    playerAttackPosition = homeAttackPositions(id, :);
    kickPower = 1;
    kickState = false;
    desiredPosition = playerAttackPosition;
    isdone = true;
  state Shoot
    en,du:
    angleBallGoal = atan2d(awayGoalPose(2) - gameSituation.ballCurrentPose(2), ...
    awayGoalPose(1) - gameSituation.ballCurrentPose(1));
    kickPower = 100;
    kickState = true;
    kickDirection = angleBallGoal;
    xPosition= gameSituation.ballCurrentPose(1) + cosd(180 - angleBallGoal) * kickableAreaRadius;
    yPosition = gameSituation.ballCurrentPose(2) + sind(180 - angleBallGoal) * kickableAreaRadius;
    desiredPosition = [xPosition, yPosition, kickDirection];
    isdone = true;
  state Pass
    en,du:
    [minval,minidx] = min(teamDistToGoal)
    angleBallPlayer = atan2d(gameSituation.robotCurrentPose(minidx, 2) - gameSituation.ballCurrentPose(2), ...
    gameSituation.robotCurrentPose(minidx, 1) - gameSituation.ballCurrentPose(1));
    kickPower = 66;
    kickState = true;
    kickDirection = angleBallPlayer;
    xPosition= gameSituation.ballCurrentPose(1) + cosd(180 - angleBallGoal) * kickableAreaRadius;
    yPosition = gameSituation.ballCurrentPose(2) + sind(180 - angleBallGoal) * kickableAreaRadius;
    desiredPosition = [xPosition, yPosition, kickDirection];
    isdone = true;
  state Dribble
    en,du:
    angleBallGoal = atan2d(awayGoalPose(2) - gameSituation.ballCurrentPose(2), ...
    awayGoalPose(1) - gameSituation.ballCurrentPose(1));
    kickPower = 10;
    %%should be designed as the kickPower = kickPowerCofficent * 100
    %%kickPowerCofficieant should also be calculated by distance
    kickState = true;
    kickDirection = angleBallGoal;
    xPosition= gameSituation.ballCurrentPose(1) + cosd(180 - angleBallGoal) * kickableAreaRadius;
    yPosition = gameSituation.ballCurrentPose(2) + sind(180 - angleBallGoal) * kickableAreaRadius;
    desiredPosition = [xPosition, yPosition, kickDirection];
    isdone = true;
  state Intercept
    en,du:
    angleBallGoal = atan2d(awayGoalPose(2) - gameSituation.ballCurrentPose(2), ...
    awayGoalPose(1) - gameSituation.ballCurrentPose(1));
    kickPower = 50;
    kickState = true;
    kickDirection = angleBallGoal;
    xPosition= gameSituation.ballCurrentPose(1) + cosd(180 - angleBallGoal) * kickableAreaRadius;
    yPosition = gameSituation.ballCurrentPose(2) + sind(180 - angleBallGoal) * kickableAreaRadius;
    desiredPosition = [xPosition, yPosition, kickDirection];
    isdone = true;
  state Formation
    en,du:
    playerDefendPosition = homeDefendPositions(id, :);
    kickPower = 1;
    kickState = false;
    desiredPosition = playerDefendPosition;
    isdone = true;
  state Kick
    state MoveTo1
      en,du:
      isdone = false;
      robotCommand.robotDestinationPose = desiredPosition;
      distToBall = distTo(gameSituation.robotCurrentPose(id,1:2), ...
      gameSituation.ballCurrentPose(1:2));
    state KickTo
      en,du:
      robotCommand.kick = kickState;
      robotCommand.kickProperty = kickPower;
      isdone = true;
    MoveTo1 -> KickTo [order 1] : [distToBall <= kickableAreaRadius+5]
  MoveTo1 -> InitialState [order 2] : [after(2,sec)]
  KickTo -> InitialState : [after(5,sec)]
  (default) -> InitialState
  InitialState -> Attack [order 2] : [gameSituation.ballLastCommandBy(1) == 2]
  InitialState -> Defend [order 1] : [gameSituation.ballLastCommandBy(1) == 1]
  Attack -> Position [order 1] : [distToBall ~= min(teamDistToBall)]
  Defend -> Intercept [order 1] : [distToBall ~= max(teamDistToBall)]
  Defend -> Formation [order 2] : [distToBall == max(teamDistToBall)]
  Attack -> Pass [order 3] : [distToGoal1 ~= min(teamDistToGoal)&& distToBall == min(teamDistToBall)]
  Attack -> Dribble [order 4] : [distToBall == min(teamDistToBall) && distToGoal1 == min(teamDistToGoal) && distToGoal1 > shootDistThres]
  Attack -> Shoot [order 2] : [distToBall == min(teamDistToBall) && distToGoal1 == min(teamDistToGoal) && distToGoal1 < shootDistThres]
  Intercept -> MoveTo1 : [isdone]
  Formation -> MoveTo1 : [isdone]
  Pass -> MoveTo1 : [isdone]
  Dribble -> MoveTo1 : [isdone]
  Shoot -> MoveTo1 : [isdone]
  Position -> MoveTo1 : [isdone]
  data: robotPosition function_input; goalPosition function_input; dist function_output; awayGoalPose local =[0 0]; homeGoalPose local =[0 0]; id local =1; idx local; angleBallGoal local =0; desiredPosition local =[0 0 0]; distToOwnGoal local =0; kickDirection local =0; kickPower local =0; kickState local =false; minidx local; playerDefendPosition local =[0 0 0]; teamDistToGoal local =[0 0 0 0]; teamDistToOwnGoal local =[0 0 0 0]; minval local; isdone local boolean =false; playerAttackPosition local =[0 0 0]; shootDistThres local =0; gameSituation input Bus: gameSituation; kickableAreaRadius local =0; distToGoal1 local =0; angleBallPlayer local =0; robotCommand output Bus: robotCommand; distToBall local =0; teamDistToBall local =[0 0 0 0]; homeAttackPositions local =[0 0 0;0 0 0;0 0 0;0 0 0]; homeDefendPositions local =[0 0 0;0 0 0;0 0 0;0 0 0]; xPosition local; yPosition local
  function dist = distTo(robotPosition,goalPosition):
    | function dist = distTo(robotPosition,goalPosition)
    |     dist = norm(robotPosition - goalPosition);
    | end

== matlab function RoboSoccerSim/Server/Subsystem1/MATLAB Function ==
  data: kickDirection output; destinationPose input
function kickDirection  = fcn(destinationPose)

kickDirection = destinationPose(3);

end

== matlab function RoboSoccerSim/Server/Subsystem1/MATLAB Function1 ==
  data: kickDirection output; destinationPose input
function kickDirection  = fcn(destinationPose)

kickDirection = destinationPose(3);

end

== matlab function RoboSoccerSim/Server/Subsystem1/MATLAB Function2 ==
  data: kickDirection output; destinationPose input
function kickDirection  = fcn(destinationPose)

kickDirection = destinationPose(3);

end

== matlab function RoboSoccerSim/Server/Subsystem1/MATLAB Function3 ==
  data: kickDirection output; destinationPose input
function kickDirection  = fcn(destinationPose)

kickDirection = destinationPose(3);

end

== matlab function RoboSoccerSim/Server/Subsystem3/MATLAB Function ==
  data: kickDirection output; destinationPose input
function kickDirection  = fcn(destinationPose)

kickDirection = destinationPose(3);

end

== matlab function RoboSoccerSim/Server/Subsystem3/MATLAB Function1 ==
  data: kickDirection output; destinationPose input
function kickDirection  = fcn(destinationPose)

kickDirection = destinationPose(3);

end

== matlab function RoboSoccerSim/Server/Subsystem3/MATLAB Function2 ==
  data: kickDirection output; destinationPose input
function kickDirection  = fcn(destinationPose)

kickDirection = destinationPose(3);

end

== matlab function RoboSoccerSim/Server/Subsystem3/MATLAB Function3 ==
  data: kickDirection output; destinationPose input
function kickDirection  = fcn(destinationPose)

kickDirection = destinationPose(3);

end
